simulink model "specificapwm"  (R2022b)
settings: Solver=VariableStepAuto  StartTime=0.0  StopTime=10.0  RelTol=1e-3
undefined symbols (not defined in the file or in its folder): pwr
libraries: simulink x2
settings Model: Creator=tborlina  LastModifiedBy=tborlina

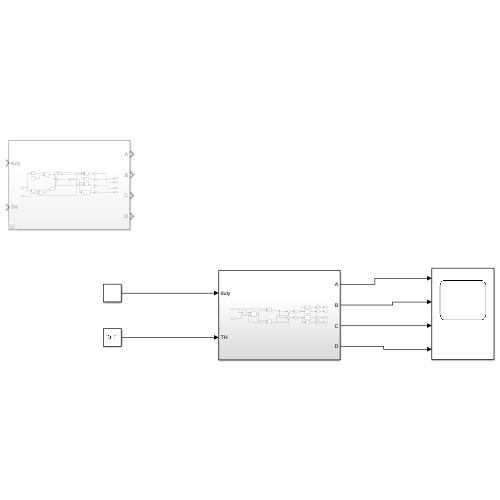
[thumbnail: Simulink's stored preview of the top-level diagram]
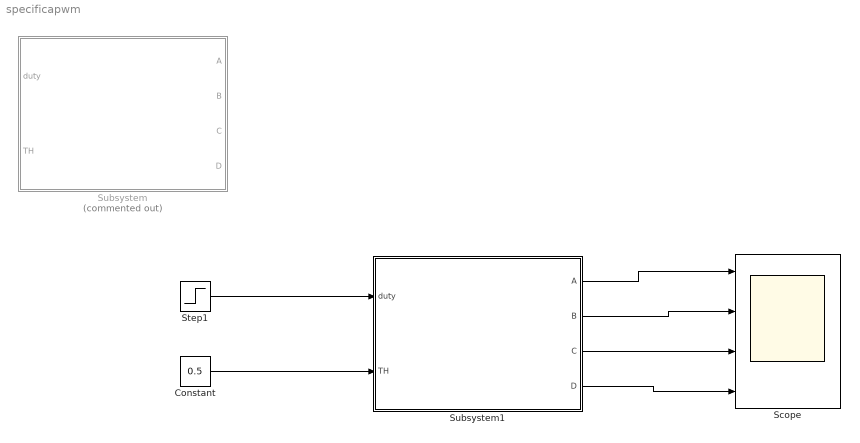
== system specificapwm ==
  Constant : Constant  Value=0.5
  Scope : Scope  NumInputPorts=4
  Step1 : Step  After=-0.75  SampleTime=0
  Subsystem : Subsystem  Commented=on
  Subsystem1 : Subsystem
  wires:
  Subsystem1/1(A) -> Scope/1
  Subsystem1/2(B) -> Scope/2
  Subsystem1/3(C) -> Scope/3
  Subsystem1/4(D) -> Scope/4
  Constant/1 -> Subsystem1/2(TH)
  Step1/1 -> Subsystem1/1(duty)

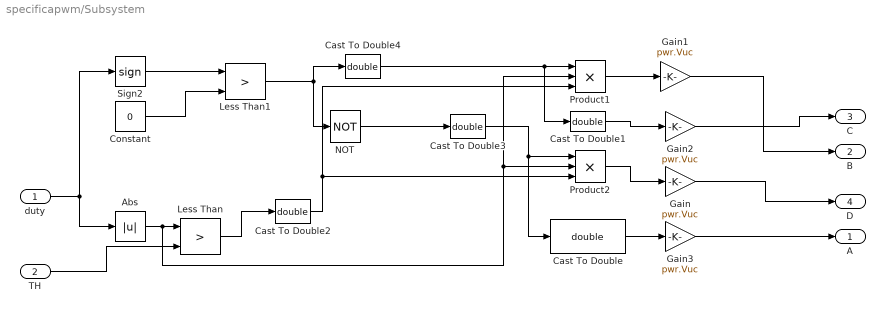
== system specificapwm/Subsystem ==
  duty : Inport
  TH : Inport  Port=2
  Abs : Abs  SaturateOnIntegerOverflow=off
  Cast To Double{,1..4} (5 alike) : DataTypeConversion  OutDataTypeStr=double  SaturateOnIntegerOverflow=off  RndMeth=Floor
  Constant : Constant  Value=0
  Gain{,1..3} (4 alike) : Gain  Gain=pwr.Vuc
  Less Than : RelationalOperator  Operator=>  OutDataTypeStr=boolean  RndMeth=Simplest  InputSameDT=off
  Less Than1 : RelationalOperator  Operator=>  OutDataTypeStr=boolean  RndMeth=Simplest  InputSameDT=off
  NOT : Logic  Operator=NOT  IconShape=distinctive  AllPortsSameDT=off  OutDataTypeStr=boolean
  Product1 : Product  Inputs=3
  Product2 : Product  Inputs=3
  Sign2 : Signum
  A : Outport
  B : Outport  Port=2
  C : Outport  Port=3
  D : Outport  Port=4
  wires:
  TH/1 -> Less Than/2
  duty/1 -> Sign2/1, Abs/1
  Less Than/1 -> Cast To Double2/1
  Sign2/1 -> Less Than1/1
  Constant/1 -> Less Than1/2
  Less Than1/1 -> NOT/1, Cast To Double4/1
  Abs/1 -> Product1/2, Product2/2, Less Than/1
  Product2/1 -> Gain/1
  Gain/1 -> D/1
  Product1/1 -> Gain1/1
  Gain1/1 -> B/1
  Gain2/1 -> C/1
  Gain3/1 -> A/1
  Cast To Double/1 -> Gain3/1
  Cast To Double1/1 -> Gain2/1
  Cast To Double2/1 -> Product2/3, Product1/3
  Cast To Double3/1 -> Cast To Double/1, Product2/1
  Cast To Double4/1 -> Cast To Double1/1, Product1/1
  NOT/1 -> Cast To Double3/1

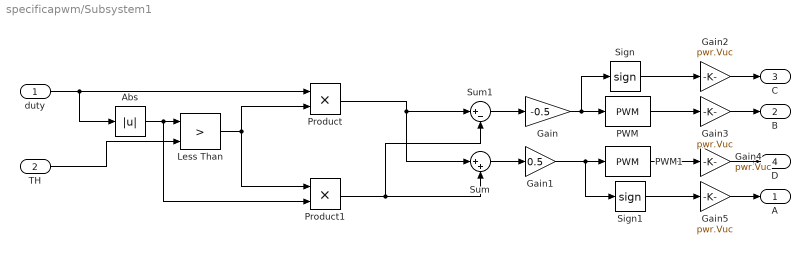
== system specificapwm/Subsystem1 ==
  duty : Inport
  TH : Inport  Port=2
  Abs : Abs  SaturateOnIntegerOverflow=off
  Gain : Gain  Gain=-0.5
  Gain1 : Gain  Gain=0.5
  Gain{2..5} (4 alike) : Gain  Gain=pwr.Vuc
  Less Than : RelationalOperator  Operator=>  OutDataTypeStr=boolean  RndMeth=Simplest  InputSameDT=off
  PWM : simulink/Discontinuities/PWM  DisableCoverage=on  Period=1  InitialDelay=0  DisallowZeroDutyCycle=off  RunAtFixedTimeIntervals=off  SampleTime=0.1
  PWM1 : simulink/Discontinuities/PWM  DisableCoverage=on  Period=1  InitialDelay=0  DisallowZeroDutyCycle=off  RunAtFixedTimeIntervals=off  SampleTime=0.1
  Product : Product
  Product1 : Product
  Sign : Signum
  Sign1 : Signum
  Sum : Sum  Inputs=|++
  Sum1 : Sum  Inputs=|+-
  A : Outport
  B : Outport  Port=2
  C : Outport  Port=3
  D : Outport  Port=4
  wires:
  Sign/1 -> Gain2/1
  Sign1/1 -> Gain5/1
  Gain1/1 -> PWM1/1, Sign1/1
  Gain/1 -> PWM/1, Sign/1
  Sum1/1 -> Gain/1
  Sum/1 -> Gain1/1
  Product1/1 -> Sum/2, Sum1/2
  Product/1 -> Sum1/1, Sum/1
  Less Than/1 -> Product1/1, Product/2
  Abs/1 -> Less Than/1, Product1/2
  duty/1 -> Product/1, Abs/1
  TH/1 -> Less Than/2
  Gain2/1 -> C/1
  Gain3/1 -> B/1
  Gain4/1 -> D/1
  Gain5/1 -> A/1
  PWM/1 -> Gain3/1
  PWM1/1 -> Gain4/1
